simulink model "MultiVehicleModel"  (R2014a)
settings: Solver=ode1  StartTime=0.0  StopTime=inf  FixedStep=simPars.SampleTime  RelTol=1e-3
undefined symbols (not defined in the file or in its folder): DiscIntNeverNeededParam, Earth, Env, eul_0, FWFleet, GVFleet, m, RCFleet, s, WGS84
undefined symbols (not defined in the file): simPars
libraries: simulink x26, aerolibtransform2 x7, instrumentlib x6, Actuator_Lib x5, aerolib6dofsys x4, etargetslib x3, aerolibasang x3, aerolibconvert2 x2, aerolibutil x1, aerolibatmos2 x1, aerolibobsolete x1, aerolibgravity2 x1
(part 3 of 4)

== system MultiVehicleModel/Reconnaissance Fleet/UMN - Uninhabited Aerial Vehicle Fleet/Nonlinear UAV Model/Environment ==
  States : Inport
  Bus Creator : BusCreator  Inputs=9
  Bus Selector1 : BusSelector  OutputSignals=Nav.Alt (Above Mean Sea Level) [m]
  Bus Selector2 : BusSelector  OutputSignals=Nav.Altitude [m],Nav.Geodetic Latitude [deg],Nav.Geodetic Longitude [deg]
  Bus Selector3 : BusSelector  OutputSignals=Nav.Geodetic Latitude [deg],Nav.Geodetic Longitude [deg],Nav.Altitude [m]  OutputAsBus=on
  Bus Selector4 : BusSelector  OutputSignals=WindAxesParam.V_s [m/s],R_be [3x3],Nav.Alt (Above Ground Level) [m]
  COESA Atmosphere Model : aerolibatmos2/COESA Atmosphere Model  units=Metric (MKS)  spec=1976 COESA-extended U.S. Standard Atmosphere  model=Profile  profile_var=High temperature  profile_percent=1%  profile_alt=5 km (16404 ft)  envelope_var=High temperature  envelope_percent=1%  action=Warning
  Constant : Constant  Value=Env.DecimalYear
  Magnetic Model : Subsystem  BlockChoice=WMM 2005
      settings: AttributesFormatString=%<BlockChoice>  TemplateBlock=Environment_Lib/Magnetic Model  MemberBlocks=WMM 2005,WMM Bypass
  README : simulink/Model-Wide Utilities/DocBlock  DocumentType=Text
      content=|
      | Environment Model
      |
      | This block uses the Aerospace Blockset models for Earth's atmosphere,
      | gravity, magnetic field, and wind.
      |
      | The atmosphere is modeled using the 1976 Standard Atmosphere block.
      |
      | Winds are modeled in two portions: steady and unsteady. The steady
      | portion is defined by a speed and direction, and is horizontal only. The
      | unsteady portion is made up of a wind gust model and a turbulence model.
      |
      | The Dryden Wind Turbulence Model is used to model turbulence. The
      | intensity of the turbulence at low altitude (<1000ft) is determined by
      | the wind speed and direction; this is set as separate variables from the
      | steady wind speed and direction. The turbulence is off by default, and
      | can be enabled by setting the Env.Winds.TurbulenceOn boolean in
      | UAV_config.m.
      |
      | The Discrete Gust Model is used to model wind gusts. Parameters are time
      | on, duration (length), and amplitude, in three axes (u,v,w). These
      | parameters are set in Env.Winds, in UAV_config.m
      |
      | Note the booleans in the Env.Winds stucture to turn on each wind
      | component: >> Env.Winds
      |
      | ans =
      |
      |      TurbulenceOn: 0
      |     TurbWindSpeed: 0
      |       TurbWindDir: 0
      |            GustOn: 0
      |     GustStartTime: 0
      |        GustLength: [1 1 1]
      |     GustAmplitude: [1 1 1]
      |      SteadyWindOn: 0
      |         WindSpeed: 0
      |           WindDir: 0
      |
      |
      | The WGS84 Gravity Model is used to model Earth's gravity as a function of
      | latitude, longitude, and altitude.
      |
      | The World Magnetic Model 2005 is used to model Earth's magnetic field as
      | a function of latitude, longitude, and altitude. The current decimal year
      | is input.
      |
      | *Note for trim/linearizing: the Dryden turbulence model and the World
      | Magnetic Model 2005 have many internal states, which makes trimming and
      | linearizing difficult. Thus "Bypass" blocks are substituted for the Winds
      | and Magnetic Model blocks using Configurable Subsystems. For the
      | UAV_NL.mdl, the block choices are automatically set to "Bypass" using the
      | models "InitFcn" callback, which can be viewed by using the Model
      | Explorer, selecting UAV_NL, and going to the "Callbacks" tab. The Nonlinear
      | UAV Model block will then show up as a Parameterized Link (red arrow in the
      | lower left corner). The SIL and PIL sims use the default blocks, and should
      | have a normal library link (black arrow).
  "WGS84 Gravity Model " : aerolibgravity2/WGS84 Gravity Model   model=WGS84 Taylor Series  units=Metric (MKS)  no_atmos=on  precessing=on  jd_loc=off  month=October  day=10  year=2004  no_centrifugal=on  action=Warning
  Winds : Subsystem  BlockChoice=Wind & Turbulence
      settings: AttributesFormatString=%<BlockChoice>  TemplateBlock=Environment_Lib/Winds  MemberBlocks=Wind & Turbulence,Wind Bypass
  EnvData : Outport
  wires:
  Constant/1 -> Magnetic Model/4(Decimal Year)
  Bus Selector3/1 -> "WGS84 Gravity Model "/1
  Bus Selector2/3 -> Magnetic Model/3(Longitude)  "<Geodetic Longitude [deg]>"
  Bus Selector2/2 -> Magnetic Model/2(Latitude)  "<Geodetic Latitude [deg]>"
  Bus Selector2/1 -> Magnetic Model/1(Altitude)  "<Altitude [m]>"
  Magnetic Model/1(Magnetic Field) -> Bus Creator/9  "Magnetic Field [nT]"
  "WGS84 Gravity Model "/1 -> Bus Creator/8  "Gravity [m/s^2]"
  Winds/3(WindAngVel [rad/s]) -> Bus Creator/7  "WindAngVel [rad/s]"
  Winds/2(WindGust [m/s]) -> Bus Creator/6  "WindGust [m/s]"
  Winds/1(SteadyWind [m/s]) -> Bus Creator/5  "SteadyWind [m/s]"
  COESA Atmosphere Model/4 -> Bus Creator/4  "Density [kg/m^3]"
  COESA Atmosphere Model/1 -> Bus Creator/1  "Temperature [K]"
  COESA Atmosphere Model/2 -> Bus Creator/2  "Speed of Sound [m/s]"
  COESA Atmosphere Model/3 -> Bus Creator/3  "Pressure [Pa]"
  States/1 -> Bus Selector1/1, Bus Selector2/1, Bus Selector3/1, Bus Selector4/1
  Bus Selector1/1 -> COESA Atmosphere Model/1  "<Alt (Above Mean Sea Level) [m]>"
  Bus Creator/1 -> EnvData/1
  Bus Selector4/1 -> Winds/1(V_s [m/s])  "<V_s [m/s]>"
  Bus Selector4/2 -> Winds/2(R_be [3x3])  "<R_be [3x3]>"
  Bus Selector4/3 -> Winds/3(h (m))  "<Alt (Above Ground Level) [m]>"

== system MultiVehicleModel/Reconnaissance Fleet/UMN - Uninhabited Aerial Vehicle Fleet/Nonlinear UAV Model/Forces and Moments ==
  Control Inputs : Inport
  States : Inport  Port=2
  EnvData : Inport  Port=3
  Aerodynamic Forces and Moments : Subsystem  AncestorBlock=Aero_Lib/Aerodynamic Forces and Moments
      mask help:
      | Set the boolean Aero Model Selection flag to 1 to use the FASER aerodynamic
      | model; otherwise, the Ultra Stick aero model will be used.
      |
      | This is done in this block's Mask Initialization commands. Also set is the
      | axes input for computing the forces and moments from the coefficients.
  Bus Selector1 : BusSelector  OutputSignals=throttle [nd]
  Control Inputs1 : InportShadow
  Electric Propulsion Forces and Moments : Propulsion_Lib/Electric Propulsion Forces and Moments
  "Gravitational Force " : Gravity_Lib/Gravitational Force 
  README : simulink/Model-Wide Utilities/DocBlock  DocumentType=Text
      content=|
      | Forces and Moments
      |
      | This block models all of the relevant external forces and
      | moments acting on the aircraft. The Aerodynamic Forces and Moments block
      | contains the aero models, and is a masked subsystem. The input parameter to
      | this block is a boolean which controls which aero model (either FASER or
      | the Ultrastick) is used.
      |
      | The Gravitational Force block models the effect of Earth's graviy field on
      | the aircraft.
      |
      | The Electric Propulsion Forces and Moments block contains the electric
      | motor model.
      |
      | Note the non-gravitational forces (nonGravForces) are output- this is what
      | an accelerometer on the aircraft would measure, and is used in the sensor
      | models.
  Sum : Sum  Inputs=+++
  Sum1 : Sum  Inputs=|++
  Sum2 : Sum  Inputs=|++
  Total Force : Outport
  Total Moment : Outport  Port=2
  nonGravForces : Outport  Port=3
  wires:
  Bus Selector1/1 -> Electric Propulsion Forces and Moments/3  "<throttle [nd]>"
  Control Inputs/1 -> Aerodynamic Forces and Moments/1(Control Surfaces)
  States/1 -> Aerodynamic Forces and Moments/2(States), "Gravitational Force "/2, Electric Propulsion Forces and Moments/2
  EnvData/1 -> Aerodynamic Forces and Moments/3(EnvData), "Gravitational Force "/1, Electric Propulsion Forces and Moments/1
  Control Inputs1/1 -> Bus Selector1/1
  Aerodynamic Forces and Moments/2(F_aero_body) -> Sum/1, Sum2/1
  "Gravitational Force "/1 -> Sum/2
  Electric Propulsion Forces and Moments/1 -> Sum2/2, Sum/3
  Sum/1 -> Total Force/1
  Aerodynamic Forces and Moments/1(M_aero_body) -> Sum1/1
  Electric Propulsion Forces and Moments/2 -> Sum1/2
  Sum1/1 -> Total Moment/1
  Sum2/1 -> nonGravForces/1

== system MultiVehicleModel/Reconnaissance Fleet/UMN - Uninhabited Aerial Vehicle Fleet/Nonlinear UAV Model/Packaging initial Euler angles  ==
  Position and heading : Inport
  Constant : Constant  Value=AC.TrimCondition.AttitudeIni(1:2)
  Demux9 : Demux  Outputs=[3 1]
  Mux : Mux  Inputs=[2 1]
  T : Terminator
  Initial Euler angles : Outport
  wires:
  Position and heading/1 -> Demux9/1
  Mux/1 -> Initial Euler angles/1
  Demux9/1 -> T/1
  Demux9/2 -> Mux/2
  Constant/1 -> Mux/1

== system MultiVehicleModel/Reconnaissance Fleet/UMN - Uninhabited Aerial Vehicle Fleet/Sensors/NoiseModel ==
  In1 : Inport
  Add : Sum  Inputs=+++
  Band-Limited White Noise : simulink/Sources/Band-Limited White Noise  Cov=sigma  Ts=timestep  seed=seed
  Gain : Gain  Gain=scf
  Gear1 : Constant  Value=bias
  Gear2 : Constant  Value=noise_on
  Noise_on : Switch  Threshold=0.5  SaturateOnIntegerOverflow=on  InputSameDT=on
  Out1 : Outport
  wires:
  In1/1 -> Gain/1, Noise_on/3
  Gain/1 -> Add/3
  Gear1/1 -> Add/2
  Add/1 -> Noise_on/1
  Band-Limited White Noise/1 -> Add/1
  Gear2/1 -> Noise_on/2
  Noise_on/1 -> Out1/1

== system MultiVehicleModel/Reconnaissance Fleet/UMN - Uninhabited Aerial Vehicle Fleet/Sensors/NoiseModel1 ==
  In1 : Inport
  Add : Sum  Inputs=+++
  Band-Limited White Noise : simulink/Sources/Band-Limited White Noise  Cov=sigma  Ts=timestep  seed=seed
  Gain : Gain  Gain=scf
  Gear1 : Constant  Value=bias
  Gear2 : Constant  Value=noise_on
  Noise_on : Switch  Threshold=0.5  SaturateOnIntegerOverflow=on  InputSameDT=on
  Out1 : Outport
  wires:
  In1/1 -> Gain/1, Noise_on/3
  Gain/1 -> Add/3
  Gear1/1 -> Add/2
  Add/1 -> Noise_on/1
  Band-Limited White Noise/1 -> Add/1
  Gear2/1 -> Noise_on/2
  Noise_on/1 -> Out1/1

== system MultiVehicleModel/Reconnaissance Fleet/UMN - Uninhabited Aerial Vehicle Fleet/Sensors/NoiseModel10 ==
  In1 : Inport
  Add : Sum  Inputs=+++
  Band-Limited White Noise : simulink/Sources/Band-Limited White Noise  Cov=sigma  Ts=timestep  seed=seed
  Gain : Gain  Gain=scf
  Gear1 : Constant  Value=bias
  Gear2 : Constant  Value=noise_on
  Noise_on : Switch  Threshold=0.5  SaturateOnIntegerOverflow=on  InputSameDT=on
  Out1 : Outport
  wires:
  In1/1 -> Gain/1, Noise_on/3
  Gain/1 -> Add/3
  Gear1/1 -> Add/2
  Add/1 -> Noise_on/1
  Band-Limited White Noise/1 -> Add/1
  Gear2/1 -> Noise_on/2
  Noise_on/1 -> Out1/1

== system MultiVehicleModel/Reconnaissance Fleet/UMN - Uninhabited Aerial Vehicle Fleet/Sensors/NoiseModel11 ==
  In1 : Inport
  Add : Sum  Inputs=+++
  Band-Limited White Noise : simulink/Sources/Band-Limited White Noise  Cov=sigma  Ts=timestep  seed=seed
  Gain : Gain  Gain=scf
  Gear1 : Constant  Value=bias
  Gear2 : Constant  Value=noise_on
  Noise_on : Switch  Threshold=0.5  SaturateOnIntegerOverflow=on  InputSameDT=on
  Out1 : Outport
  wires:
  In1/1 -> Gain/1, Noise_on/3
  Gain/1 -> Add/3
  Gear1/1 -> Add/2
  Add/1 -> Noise_on/1
  Band-Limited White Noise/1 -> Add/1
  Gear2/1 -> Noise_on/2
  Noise_on/1 -> Out1/1

== system MultiVehicleModel/Reconnaissance Fleet/UMN - Uninhabited Aerial Vehicle Fleet/Sensors/NoiseModel12 ==
  In1 : Inport
  Add : Sum  Inputs=+++
  Band-Limited White Noise : simulink/Sources/Band-Limited White Noise  Cov=sigma  Ts=timestep  seed=seed
  Gain : Gain  Gain=scf
  Gear1 : Constant  Value=bias
  Gear2 : Constant  Value=noise_on
  Noise_on : Switch  Threshold=0.5  SaturateOnIntegerOverflow=on  InputSameDT=on
  Out1 : Outport
  wires:
  In1/1 -> Gain/1, Noise_on/3
  Gain/1 -> Add/3
  Gear1/1 -> Add/2
  Add/1 -> Noise_on/1
  Band-Limited White Noise/1 -> Add/1
  Gear2/1 -> Noise_on/2
  Noise_on/1 -> Out1/1

== system MultiVehicleModel/Reconnaissance Fleet/UMN - Uninhabited Aerial Vehicle Fleet/Sensors/NoiseModel2 ==
  In1 : Inport
  Add : Sum  Inputs=+++
  Band-Limited White Noise : simulink/Sources/Band-Limited White Noise  Cov=sigma  Ts=timestep  seed=seed
  Gain : Gain  Gain=scf
  Gear1 : Constant  Value=bias
  Gear2 : Constant  Value=noise_on
  Noise_on : Switch  Threshold=0.5  SaturateOnIntegerOverflow=on  InputSameDT=on
  Out1 : Outport
  wires:
  In1/1 -> Gain/1, Noise_on/3
  Gain/1 -> Add/3
  Gear1/1 -> Add/2
  Add/1 -> Noise_on/1
  Band-Limited White Noise/1 -> Add/1
  Gear2/1 -> Noise_on/2
  Noise_on/1 -> Out1/1

== system MultiVehicleModel/Reconnaissance Fleet/UMN - Uninhabited Aerial Vehicle Fleet/Sensors/NoiseModel3 ==
  In1 : Inport
  Add : Sum  Inputs=+++
  Band-Limited White Noise : simulink/Sources/Band-Limited White Noise  Cov=sigma  Ts=timestep  seed=seed
  Gain : Gain  Gain=scf
  Gear1 : Constant  Value=bias
  Gear2 : Constant  Value=noise_on
  Noise_on : Switch  Threshold=0.5  SaturateOnIntegerOverflow=on  InputSameDT=on
  Out1 : Outport
  wires:
  In1/1 -> Gain/1, Noise_on/3
  Gain/1 -> Add/3
  Gear1/1 -> Add/2
  Add/1 -> Noise_on/1
  Band-Limited White Noise/1 -> Add/1
  Gear2/1 -> Noise_on/2
  Noise_on/1 -> Out1/1

== system MultiVehicleModel/Reconnaissance Fleet/UMN - Uninhabited Aerial Vehicle Fleet/Sensors/NoiseModel4 ==
  In1 : Inport
  Add : Sum  Inputs=+++
  Band-Limited White Noise : simulink/Sources/Band-Limited White Noise  Cov=sigma  Ts=timestep  seed=seed
  Gain : Gain  Gain=scf
  Gear1 : Constant  Value=bias
  Gear2 : Constant  Value=noise_on
  Noise_on : Switch  Threshold=0.5  SaturateOnIntegerOverflow=on  InputSameDT=on
  Out1 : Outport
  wires:
  In1/1 -> Gain/1, Noise_on/3
  Gain/1 -> Add/3
  Gear1/1 -> Add/2
  Add/1 -> Noise_on/1
  Band-Limited White Noise/1 -> Add/1
  Gear2/1 -> Noise_on/2
  Noise_on/1 -> Out1/1

== system MultiVehicleModel/Reconnaissance Fleet/UMN - Uninhabited Aerial Vehicle Fleet/Sensors/NoiseModel5 ==
  In1 : Inport
  Add : Sum  Inputs=+++
  Band-Limited White Noise : simulink/Sources/Band-Limited White Noise  Cov=sigma  Ts=timestep  seed=seed
  Gain : Gain  Gain=scf
  Gear1 : Constant  Value=bias
  Gear2 : Constant  Value=noise_on
  Noise_on : Switch  Threshold=0.5  SaturateOnIntegerOverflow=on  InputSameDT=on
  Out1 : Outport
  wires:
  In1/1 -> Gain/1, Noise_on/3
  Gain/1 -> Add/3
  Gear1/1 -> Add/2
  Add/1 -> Noise_on/1
  Band-Limited White Noise/1 -> Add/1
  Gear2/1 -> Noise_on/2
  Noise_on/1 -> Out1/1

== system MultiVehicleModel/Reconnaissance Fleet/UMN - Uninhabited Aerial Vehicle Fleet/Sensors/NoiseModel6 ==
  In1 : Inport
  Add : Sum  Inputs=+++
  Band-Limited White Noise : simulink/Sources/Band-Limited White Noise  Cov=sigma  Ts=timestep  seed=seed
  Gain : Gain  Gain=scf
  Gear1 : Constant  Value=bias
  Gear2 : Constant  Value=noise_on
  Noise_on : Switch  Threshold=0.5  SaturateOnIntegerOverflow=on  InputSameDT=on
  Out1 : Outport
  wires:
  In1/1 -> Gain/1, Noise_on/3
  Gain/1 -> Add/3
  Gear1/1 -> Add/2
  Add/1 -> Noise_on/1
  Band-Limited White Noise/1 -> Add/1
  Gear2/1 -> Noise_on/2
  Noise_on/1 -> Out1/1

== system MultiVehicleModel/Reconnaissance Fleet/UMN - Uninhabited Aerial Vehicle Fleet/Sensors/NoiseModel7 ==
  In1 : Inport
  Add : Sum  Inputs=+++
  Band-Limited White Noise : simulink/Sources/Band-Limited White Noise  Cov=sigma  Ts=timestep  seed=seed
  Gain : Gain  Gain=scf
  Gear1 : Constant  Value=bias
  Gear2 : Constant  Value=noise_on
  Noise_on : Switch  Threshold=0.5  SaturateOnIntegerOverflow=on  InputSameDT=on
  Out1 : Outport
  wires:
  In1/1 -> Gain/1, Noise_on/3
  Gain/1 -> Add/3
  Gear1/1 -> Add/2
  Add/1 -> Noise_on/1
  Band-Limited White Noise/1 -> Add/1
  Gear2/1 -> Noise_on/2
  Noise_on/1 -> Out1/1

== system MultiVehicleModel/Reconnaissance Fleet/UMN - Uninhabited Aerial Vehicle Fleet/Sensors/NoiseModel8 ==
  In1 : Inport
  Add : Sum  Inputs=+++
  Band-Limited White Noise : simulink/Sources/Band-Limited White Noise  Cov=sigma  Ts=timestep  seed=seed
  Gain : Gain  Gain=scf
  Gear1 : Constant  Value=bias
  Gear2 : Constant  Value=noise_on
  Noise_on : Switch  Threshold=0.5  SaturateOnIntegerOverflow=on  InputSameDT=on
  Out1 : Outport
  wires:
  In1/1 -> Gain/1, Noise_on/3
  Gain/1 -> Add/3
  Gear1/1 -> Add/2
  Add/1 -> Noise_on/1
  Band-Limited White Noise/1 -> Add/1
  Gear2/1 -> Noise_on/2
  Noise_on/1 -> Out1/1

== system MultiVehicleModel/Reconnaissance Fleet/UMN - Uninhabited Aerial Vehicle Fleet/Sensors/NoiseModel9 ==
  In1 : Inport
  Add : Sum  Inputs=+++
  Band-Limited White Noise : simulink/Sources/Band-Limited White Noise  Cov=sigma  Ts=timestep  seed=seed
  Gain : Gain  Gain=scf
  Gear1 : Constant  Value=bias
  Gear2 : Constant  Value=noise_on
  Noise_on : Switch  Threshold=0.5  SaturateOnIntegerOverflow=on  InputSameDT=on
  Out1 : Outport
  wires:
  In1/1 -> Gain/1, Noise_on/3
  Gain/1 -> Add/3
  Gear1/1 -> Add/2
  Add/1 -> Noise_on/1
  Band-Limited White Noise/1 -> Add/1
  Gear2/1 -> Noise_on/2
  Noise_on/1 -> Out1/1

== system MultiVehicleModel/Rotorcraft fleet/Multiple Rotorcraft/Guidance /From geodetic to NED coordinate representation ==
  geodetic [lat,lon,alt] : Inport  Partition=on  PartitionDimension=2  PartitionWidth=1
  Demux : Demux  Outputs=[2 1]
  For Each : ForEach  DisableCoverage=on  IndexMode=One-based
  Ground Height1 : Constant  Value=Env.GroundAlt
  LLA to Flat Earth : aerolibtransform2/LLA to Flat Earth  units=Metric (MKS)  ptype=Earth (WGS84)  F=1/298.257223563  R=6378137  LL0=RCFleet.IC.geodetic(1:2)  psi=0
  "[N,E,D] (m)" : Outport  ConcatenationDimension=2
  wires:
  LLA to Flat Earth/1 -> "[N,E,D] (m)"/1
  Demux/1 -> LLA to Flat Earth/1
  Demux/2 -> LLA to Flat Earth/2
  geodetic [lat,lon,alt]/1 -> Demux/1
  Ground Height1/1 -> LLA to Flat Earth/3

== system MultiVehicleModel/Rotorcraft fleet/Multiple Rotorcraft/Navigation/EGM-96 Geoid Model ==
  Position : Inport
  Demux2 : Demux  Outputs=3
  Look-Up Table (2-D) : Lookup2D  RowIndex=Lat  ColumnIndex=Lon  Table=Alterr'  SaturateOnIntegerOverflow=on  InputSameDT=on
  Sum : Sum  Inputs=|+++
  WGS-84 correction : Constant  Value=-0.53
  MSLAlt : Outport
  wires:
  Demux2/2 -> Look-Up Table (2-D)/2
  Demux2/1 -> Look-Up Table (2-D)/1
  Position/1 -> Demux2/1
  Demux2/3 -> Sum/2
  Sum/1 -> MSLAlt/1
  Look-Up Table (2-D)/1 -> Sum/1
  WGS-84 correction/1 -> Sum/3

== system MultiVehicleModel/Rotorcraft fleet/Multiple Rotorcraft/Navigation/Ground Detection ==
  MSLAlt : Inport
  GndAlt : Inport  Port=2
  False : Constant  Value=0
  Sum : Sum  Inputs=|+-  SaturateOnIntegerOverflow=on  InputSameDT=on  OutDataTypeStr=Inherit: Same as first input
  Switch : Switch  SaturateOnIntegerOverflow=on  InputSameDT=on
  True : Constant
  AConGnd : Outport
  AGLAlt : Outport  Port=2
  wires:
  MSLAlt/1 -> Sum/1
  GndAlt/1 -> Sum/2
  Sum/1 -> Switch/2, AGLAlt/1
  False/1 -> Switch/1
  True/1 -> Switch/3
  Switch/1 -> AConGnd/1

== system MultiVehicleModel/Rotorcraft fleet/Multiple Rotorcraft/Navigation/Latitude Bound [-180,180] ==
  In : Inport
  2pi : Constant  Value=360
  Math Function : Math  Operator=mod  SaturateOnIntegerOverflow=on
  Sum1 : Sum  Inputs=|+-  SaturateOnIntegerOverflow=on  InputSameDT=on  OutDataTypeStr=Inherit: Same as first input
  Sum2 : Sum  Inputs=|++  SaturateOnIntegerOverflow=on  InputSameDT=on  OutDataTypeStr=Inherit: Same as first input
  pi : Constant  Value=180
  Out : Outport
  wires:
  Math Function/1 -> Sum1/1
  2pi/1 -> Math Function/2
  In/1 -> Sum2/1
  Sum2/1 -> Math Function/1
  pi/1 -> Sum2/2, Sum1/2
  Sum1/1 -> Out/1

== system MultiVehicleModel/Rotorcraft fleet/Multiple Rotorcraft/Navigation/Longitude Bound 0-360 ==
  In : Inport
  2pi : Constant  Value=360
  Math Function : Math  Operator=mod  SaturateOnIntegerOverflow=on
  Out : Outport
  wires:
  Math Function/1 -> Out/1
  2pi/1 -> Math Function/2
  In/1 -> Math Function/1

== system MultiVehicleModel/Reconnaissance Fleet/UMN - Uninhabited Aerial Vehicle Fleet/Control System/Control_Algorithm /Altitude Tracker ==
  h_cmd [m/s] : Inport
  h [m] : Inport  Port=2
  Altitude Tracker : Subsystem
  Discrete Transfer Fcn : DiscreteTransferFcn  Numerator=[control.LP_filter(1,2)]  Denominator=[1 control.LP_filter(2,2)]  InitialStates=OperatingPoint.op_report.Outputs(4).y/control.LP_filter(1,2)  SampleTime=SampleTime
  Saturation : Saturate  UpperLimit=control.theta_sat*pi/180  LowerLimit=-control.theta_sat*pi/180  SampleTime=SampleTime
  Sum4 : Sum  Inputs=|+-  SampleTime=SampleTime
  Sum5 : Sum  Inputs=|+-  SampleTime=SampleTime
  trim altitude : Constant  Value=OperatingPoint.op_report.Outputs(4).y
  theta_cmd [rad] : Outport
  wires:
  h_cmd [m/s]/1 -> Sum4/1
  trim altitude/1 -> Sum5/2
  Sum5/1 -> Sum4/2
  h [m]/1 -> Discrete Transfer Fcn/1
  Discrete Transfer Fcn/1 -> Sum5/1
  Sum4/1 -> Altitude Tracker/2(error)
  Altitude Tracker/1(h_out) -> Saturation/1, Altitude Tracker/1(" h_out")
  Saturation/1 -> theta_cmd [rad]/1

== system MultiVehicleModel/Reconnaissance Fleet/UMN - Uninhabited Aerial Vehicle Fleet/Control System/Control_Algorithm /Velocity Tracker ==
  V_cmd [m/s] : Inport
  V_s [m/s] : Inport  Port=2
  "    " : Constant  Value=TrimCondition.WindAxesIni(1)
  Anti Windup : Actuator_Lib/Anti Windup  MAX_DEF=AC.Actuator.throttle.PosLim-TrimCondition.Inputs.throttle  MIN_DEF=AC.Actuator.throttle.NegLim-TrimCondition.Inputs.throttle  gain_sign=on
  Discrete Transfer Fcn : DiscreteTransferFcn  Numerator=[control.LP_filter(1,2)]  Denominator=[1 control.LP_filter(2,2)]  InitialStates=TrimCondition.target.V_s/control.LP_filter(1,2)  SampleTime=SampleTime
  Discrete-Time Integrator : DiscreteIntegrator  SampleTime=.02  ICPrevOutput=DiscIntNeverNeededParam  ICPrevScaledInput=DiscIntNeverNeededParam
  Gain : Gain  Gain=control.kp_VT
  Gain1 : Gain  Gain=control.ki_VT
  Saturation1 : Saturate  UpperLimit=AC.Actuator.throttle.PosLim-TrimCondition.Inputs.throttle  LowerLimit=AC.Actuator.throttle.NegLim-TrimCondition.Inputs.throttle  SampleTime=SampleTime
  Sum : Sum  Inputs=|++
  Sum1 : Sum  Inputs=|+-
  Sum5 : Sum  Inputs=|+-  SampleTime=SampleTime
  "Throttle " : Outport
  wires:
  Discrete-Time Integrator/1 -> Gain1/1
  Gain1/1 -> Sum/1
  Gain/1 -> Sum/2
  V_cmd [m/s]/1 -> Sum1/1
  Sum/1 -> Saturation1/1, Anti Windup/1
  "    "/1 -> Sum5/2
  Sum5/1 -> Sum1/2
  V_s [m/s]/1 -> Discrete Transfer Fcn/1
  Saturation1/1 -> "Throttle "/1
  Sum1/1 -> Anti Windup/2, Gain/1
  Anti Windup/1 -> Discrete-Time Integrator/1
  Discrete Transfer Fcn/1 -> Sum5/1

== system MultiVehicleModel/Reconnaissance Fleet/UMN - Uninhabited Aerial Vehicle Fleet/Control System/Control_Algorithm /baseline control ==
  theta_cmd [rad] : Inport
  theta [rad] : Inport  Port=2
  q [rad/sec] : Inport  Port=3
  r [rad/sec] : Inport  Port=4
  phi_cmd [rad] : Inport  Port=5
  phi [rad] : Inport  Port=6
  p [rad/sec] : Inport  Port=7
  Phi Tracker : Subsystem
  Theta Tracker : Subsystem
  Yaw Damper : Subsystem
  elevator [rad] : Outport
  rudder [rad] : Outport  Port=2
  aileron [rad] : Outport  Port=3
  wires:
  p [rad/sec]/1 -> Phi Tracker/3(p [rad])
  phi [rad]/1 -> Phi Tracker/2(phi [rad])
  phi_cmd [rad]/1 -> Phi Tracker/1(phi_cmd [rad])
  Phi Tracker/1(aileron [rad]) -> aileron [rad]/1
  r [rad/sec]/1 -> Yaw Damper/1(r [rad/sec])
  Yaw Damper/1(rudder [rad]) -> rudder [rad]/1
  Theta Tracker/1(elevator [rad]) -> elevator [rad]/1
  q [rad/sec]/1 -> Theta Tracker/3(q [rad/sec])
  theta [rad]/1 -> Theta Tracker/2(theta [rad])
  theta_cmd [rad]/1 -> Theta Tracker/1(theta_cmd [rad/s])

== system MultiVehicleModel/Reconnaissance Fleet/UMN - Uninhabited Aerial Vehicle Fleet/Control System/Control_Algorithm /ground trak angle control law ==
  ground track reference angle (rad) : Inport
  heading angle (rad) : Inport  Port=2
  Saturation : Saturate  UpperLimit=40*pi/180  LowerLimit=-40*pi/180
  Sum : Sum  Inputs=|+-
  normalize angle between pi and -pi (rad) : MATLAB Function  TreatAsAtomicUnit=on
  proportional control : Gain
  phi cmd (rad) : Outport
  wires:
  ground track reference angle (rad)/1 -> Sum/1
  normalize angle between pi and -pi (rad)/1(angleOut) -> proportional control/1
  heading angle (rad)/1 -> Sum/2
  Sum/1 -> normalize angle between pi and -pi (rad)/1(angleIn)
  Saturation/1 -> phi cmd (rad)/1
  proportional control/1 -> Saturation/1

== system MultiVehicleModel/Reconnaissance Fleet/UMN - Uninhabited Aerial Vehicle Fleet/Guidance algorithm/From geodetic to NED coordinate representation/EGM-96 Geoid Model ==
  Position : Inport
  Demux2 : Demux  Outputs=3
  Look-Up Table (2-D) : Lookup2D  RowIndex=Lat  ColumnIndex=Lon  Table=Alterr'  SaturateOnIntegerOverflow=on  InputSameDT=on
  Sum : Sum  Inputs=|+++
  WGS-84 correction : Constant  Value=-0.53
  MSLAlt : Outport
  wires:
  Demux2/2 -> Look-Up Table (2-D)/2
  Demux2/1 -> Look-Up Table (2-D)/1
  Position/1 -> Demux2/1
  Demux2/3 -> Sum/2
  Sum/1 -> MSLAlt/1
  Look-Up Table (2-D)/1 -> Sum/1
  WGS-84 correction/1 -> Sum/3

== system MultiVehicleModel/Reconnaissance Fleet/UMN - Uninhabited Aerial Vehicle Fleet/Guidance algorithm/From geodetic to NED coordinate representation/Ground Detection ==
  MSLAlt : Inport
  GndAlt : Inport  Port=2
  False : Constant  Value=0
  Sum : Sum  Inputs=|+-  SaturateOnIntegerOverflow=on  InputSameDT=on  OutDataTypeStr=Inherit: Same as first input
  Switch : Switch  SaturateOnIntegerOverflow=on  InputSameDT=on
  True : Constant
  AConGnd : Outport
  AGLAlt : Outport  Port=2
  wires:
  MSLAlt/1 -> Sum/1
  GndAlt/1 -> Sum/2
  Sum/1 -> Switch/2, AGLAlt/1
  False/1 -> Switch/1
  True/1 -> Switch/3
  Switch/1 -> AConGnd/1

== system MultiVehicleModel/Reconnaissance Fleet/UMN - Uninhabited Aerial Vehicle Fleet/Guidance algorithm/From geodetic to NED coordinate representation/Latitude Bound [-180,180] ==
  In : Inport
  2pi : Constant  Value=360
  Math Function : Math  Operator=mod  SaturateOnIntegerOverflow=on
  Sum1 : Sum  Inputs=|+-  SaturateOnIntegerOverflow=on  InputSameDT=on  OutDataTypeStr=Inherit: Same as first input
  Sum2 : Sum  Inputs=|++  SaturateOnIntegerOverflow=on  InputSameDT=on  OutDataTypeStr=Inherit: Same as first input
  pi : Constant  Value=180
  Out : Outport
  wires:
  Math Function/1 -> Sum1/1
  2pi/1 -> Math Function/2
  In/1 -> Sum2/1
  Sum2/1 -> Math Function/1
  pi/1 -> Sum2/2, Sum1/2
  Sum1/1 -> Out/1

== system MultiVehicleModel/Reconnaissance Fleet/UMN - Uninhabited Aerial Vehicle Fleet/Guidance algorithm/From geodetic to NED coordinate representation/Longitude Bound 0-360 ==
  In : Inport
  2pi : Constant  Value=360
  Math Function : Math  Operator=mod  SaturateOnIntegerOverflow=on
  Out : Outport
  wires:
  Math Function/1 -> Out/1
  2pi/1 -> Math Function/2
  In/1 -> Math Function/1

== system MultiVehicleModel/Reconnaissance Fleet/UMN - Uninhabited Aerial Vehicle Fleet/Nonlinear UAV Model/6DoF EOM/calculate DCM and Euler angles ==
  "p q r " : Inport
  euler ini. (rad) : Inport  Port=2
  Rotation Angles to Direction Cosine Matrix : aerolibtransform2/Rotation Angles to Direction Cosine Matrix  rotationOrder=ZYX
  Selector : Selector  InputPortWidth=3  Indices=[3 2 1]
  phi theta psi : Integrator  InitialConditionSource=external  InitialCondition=eul_0
  phidot thetadot psidot : aerolib6dofsys/DCM & Euler Angles (Euler)/phidot thetadot psidot
  DCM1 : Outport
  Euler1 : Outport  Port=2
  wires:
  Selector/1 -> Rotation Angles to Direction Cosine Matrix/1
  phidot thetadot psidot/1 -> phi theta psi/1
  phi theta psi/1 -> Selector/1, Euler1/1, phidot thetadot psidot/2
  Rotation Angles to Direction Cosine Matrix/1 -> DCM1/1
  "p q r "/1 -> phidot thetadot psidot/1
  euler ini. (rad)/1 -> phi theta psi/2

== system MultiVehicleModel/Reconnaissance Fleet/UMN - Uninhabited Aerial Vehicle Fleet/Nonlinear UAV Model/6DoF EOM/transform to Inertial axes  ==
  x y z : Inport
  transform coefficients : Inport  Port=2
  Product : Product  Multiplication=Matrix(*)  SaturateOnIntegerOverflow=on  InputSameDT=on  OutDataTypeStr=Inherit: Same as first input
  Reshape1 : Reshape  OutputDimensionality=Column vector (2-D)
  Reshape2 : Reshape
  Ve : Outport
  wires:
  Product/1 -> Reshape2/1
  transform coefficients/1 -> Product/1
  x y z/1 -> Reshape1/1
  Reshape1/1 -> Product/2
  Reshape2/1 -> Ve/1

== system MultiVehicleModel/Reconnaissance Fleet/UMN - Uninhabited Aerial Vehicle Fleet/Nonlinear UAV Model/Auxiliary Equations/Euler Angle Bounds ==
  Euler_nobound : Inport
  2pi Bound : Subsystem
  Demux : Demux  Outputs=3
  Mux : Mux  Inputs=3
  pi Bound : Subsystem
  pi/2 Bound : Subsystem
  Euler_bound : Outport
  wires:
  2pi Bound/1(Out) -> Mux/3
  Demux/3 -> 2pi Bound/1(In)
  Demux/2 -> pi Bound/1(In)
  Demux/1 -> pi/2 Bound/1(In)
  Euler_nobound/1 -> Demux/1
  Mux/1 -> Euler_bound/1
  pi/2 Bound/1(Out) -> Mux/1
  pi Bound/1(Out) -> Mux/2

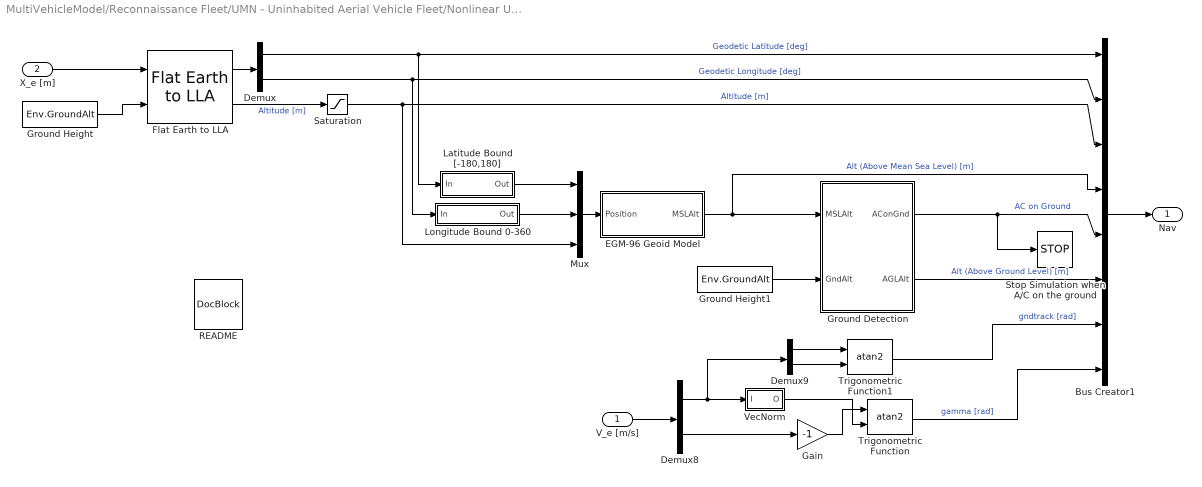
== system MultiVehicleModel/Reconnaissance Fleet/UMN - Uninhabited Aerial Vehicle Fleet/Nonlinear UAV Model/Auxiliary Equations/Navigation ==
  V_e [m/s] : Inport
  X_e [m] : Inport  Port=2
  Bus Creator1 : BusCreator  Inputs=8
  Demux : Demux  Outputs=2
  Demux8 : Demux  Outputs=[2 1]
  Demux9 : Demux  Outputs=2
  EGM-96 Geoid Model : Subsystem  mask(EGM-96 geoid undulation model){}
      mask help: Computes the MSL (mean sea level) altitude as a function of position.
      mask init:
      | load('egm96');
      mask Help:
      | The block computes the mean-sea-level altitude relative to the WGS-84 geoid.
      | <P><B>Inputs:</B>
      | <LI>Position = the 3x1 vector of aircraft location [Latitude Longitude Altitude], in [rad rad m]</LI>
      | </P>
      | <P><B>Output:</B>
      | <LI>MSLAlt = the mean-sea-level altitude, in m</LI>
      | </P>
  Flat Earth to LLA : aerolibtransform2/Flat Earth to LLA  units=Metric (MKS)  ptype=Earth (WGS84)  F=1/298.257223563  R=6378137  LL0=FWFleet.IC.geodetic(1:2)  psi=0
  Gain : Gain  Gain=-1
  Ground Detection : Subsystem  mask(Ground detection){}
      mask help: Computes altitude above ground and sets a flag if AGL is negative.
      mask Help:
      | The block computes the altitude above ground (AGL) and sets a flag if the AGL is negative (used for ground contact detection).
      | <P><B>Inputs:</B>
      | <LI>MSLAlt = the altitude measured from mean-sea-level, in meters</LI>
      | <LI>GndAlt = the altitude of the terrain (above MSL) at current location, in meters</LI>
      | </P>
      | <P><B>Output:</B>
      | <LI>AConGnd = the aircraft-on-ground flag (0 if aircraft above ground, 1 if aircraft on the ground)</LI>
      | <LI>AGLAlt = the altitude of the aircraft above ground</LI>
      | </P>
  Ground Height : Constant  Value=Env.GroundAlt
  Ground Height1 : Constant  Value=Env.GroundAlt
  Latitude Bound [-180,180] : Subsystem
  Longitude Bound 0-360 : Subsystem  mask(Longitude bound){}
      mask help: Bounds the longitude to [0, 2pi]. When 0 bound is exceeded the longitude wraps back to 2pi; when the 2pi bound is exceeded the longitude wraps back to 0.
  Mux : Mux  Inputs=3
  README : simulink/Model-Wide Utilities/DocBlock  DocumentType=Text
      content=|
      | Navigation
      |
      | This block is library link that contains the navigational model and
      | equations. Included are equations relating the flat Earth position to
      | latitude/longitude, a simplified 2D table lookup version of the EGM-96
      | Geoid model for computation of MSL/AGL altitudes, and computation of
      | flight path and ground track angles.
  Saturation : Saturate  UpperLimit=Inf  LowerLimit=0
  Stop Simulation when A/C on the ground : Stop
  Trigonometric Function : Trigonometry  Operator=atan2
  Trigonometric Function1 : Trigonometry  Operator=atan2
  VecNorm : Subsystem
  Nav : Outport
  wires:
  Gain/1 -> Trigonometric Function/1
  Demux9/1 -> Trigonometric Function1/1
  Demux8/1 -> Demux9/1, VecNorm/1(I)
  Trigonometric Function1/1 -> Bus Creator1/7  "gndtrack [rad]"
  Demux9/2 -> Trigonometric Function1/2
  Trigonometric Function/1 -> Bus Creator1/8  "gamma [rad]"
  VecNorm/1(O) -> Trigonometric Function/2
  Demux8/2 -> Gain/1
  V_e [m/s]/1 -> Demux8/1
  Ground Detection/2(AGLAlt) -> Bus Creator1/6  "Alt (Above Ground Level) [m]"
  Saturation/1 -> Mux/3, Bus Creator1/3  "Altitude [m]"
  Ground Detection/1(AConGnd) -> Stop Simulation when A/C on the ground/1, Bus Creator1/5  "AC on Ground"
  Ground Height1/1 -> Ground Detection/2(GndAlt)
  EGM-96 Geoid Model/1(MSLAlt) -> Bus Creator1/4, Ground Detection/1(MSLAlt)  "Alt (Above Mean Sea Level) [m]"
  Bus Creator1/1 -> Nav/1
  Ground Height/1 -> Flat Earth to LLA/2
  X_e [m]/1 -> Flat Earth to LLA/1
  Demux/2 -> Longitude Bound 0-360/1(In), Bus Creator1/2  "Geodetic Longitude [deg]"
  Demux/1 -> Bus Creator1/1, Latitude Bound [-180,180]/1(In)  "Geodetic Latitude [deg]"
  Flat Earth to LLA/2 -> Saturation/1  "Altitude [m]"
  Flat Earth to LLA/1 -> Demux/1
  Mux/1 -> EGM-96 Geoid Model/1(Position)
  Longitude Bound 0-360/1(Out) -> Mux/2
  Latitude Bound [-180,180]/1(Out) -> Mux/1

== system MultiVehicleModel/Reconnaissance Fleet/UMN - Uninhabited Aerial Vehicle Fleet/Nonlinear UAV Model/Environment/Magnetic Model ==
  Altitude : Inport
  Latitude : Inport  Port=2
  Longitude : Inport  Port=3
  Decimal Year : Inport  Port=4
  WMM 2005 : aerolibobsolete/World Magnetic Model 2005  units=Metric (MKS)  time_in=off  month=August  day=1  year=2009  action=None  h_out=off  dec_out=off  inc_out=off  ti_out=off
  term4 : Terminator
  Magnetic Field : Outport
  wires:
  Altitude/1 -> WMM 2005/1
  Latitude/1 -> WMM 2005/2
  Longitude/1 -> WMM 2005/3
  WMM 2005/1 -> Magnetic Field/1
  Decimal Year/1 -> term4/1

== system MultiVehicleModel/Reconnaissance Fleet/UMN - Uninhabited Aerial Vehicle Fleet/Nonlinear UAV Model/Environment/Winds ==
  V_s [m/s] : Inport
  R_be [3x3] : Inport  Port=2
  h (m) : Inport  Port=3
  Wind & Turbulence : Environment_Lib/Wind & Turbulence
  SteadyWind [m/s] : Outport
  WindGust [m/s] : Outport  Port=2
  WindAngVel [rad/s] : Outport  Port=3
  wires:
  V_s [m/s]/1 -> Wind & Turbulence/1
  R_be [3x3]/1 -> Wind & Turbulence/2
  h (m)/1 -> Wind & Turbulence/3
  Wind & Turbulence/1 -> SteadyWind [m/s]/1
  Wind & Turbulence/2 -> WindGust [m/s]/1
  Wind & Turbulence/3 -> WindAngVel [rad/s]/1

== system MultiVehicleModel/Reconnaissance Fleet/UMN - Uninhabited Aerial Vehicle Fleet/Nonlinear UAV Model/Forces and Moments/Aerodynamic Forces and Moments ==
  Control Surfaces : Inport
  States : Inport  Port=2
  EnvData : Inport  Port=3
  Bus Selector : BusSelector  OutputSignals=Density [kg/m^3]
  Bus Selector1 : BusSelector  OutputSignals=V_b [m/s]
  CG Position : Constant  Value=AC.Geometry.rCG
  CP Position : Constant  Value=AC.Geometry.AeroCenter
  Dynamic Pressure : aerolibasang/Dynamic Pressure
  "Forces and Moments Calculation " : aerolibadyn/Aerodynamic Forces and Moments   inputAxes=Wind  outputForceAxes=Body  outputMomentAxes=Wind  S=AC.Geometry.S  b=AC.Geometry.b  cbar=AC.Geometry.c
  Ultrastick : Ultrastick_Aero_Lib/Ultrastick
  M_aero_body : Outport
  F_aero_body : Outport  Port=2
  wires:
  Control Surfaces/1 -> Ultrastick/1
  Dynamic Pressure/1 -> "Forces and Moments Calculation "/2
  "Forces and Moments Calculation "/2 -> M_aero_body/1
  "Forces and Moments Calculation "/1 -> F_aero_body/1
  Bus Selector/1 -> Dynamic Pressure/2  "<Density [kg/m^3]>"
  States/1 -> Ultrastick/2, Bus Selector1/1
  EnvData/1 -> Bus Selector/1
  CP Position/1 -> "Forces and Moments Calculation "/4
  CG Position/1 -> "Forces and Moments Calculation "/3
  Ultrastick/1 -> "Forces and Moments Calculation "/1
  Bus Selector1/1 -> Dynamic Pressure/1, "Forces and Moments Calculation "/5  "<V_b [m/s]>"

== system MultiVehicleModel/Reconnaissance Fleet/UMN - Uninhabited Aerial Vehicle Fleet/Control System/Control_Algorithm /Altitude Tracker/Altitude Tracker ==
  " h_out" : Inport
  error : Inport  Port=2
  Anti Windup : Actuator_Lib/Anti Windup  MAX_DEF=AC.Actuator.elevator.PosLim-TrimCondition.Inputs.elevator  MIN_DEF=AC.Actuator.elevator.NegLim-TrimCondition.Inputs.elevator  gain_sign=on
  Discrete-Time Integrator : DiscreteIntegrator  SampleTime=.02  ICPrevOutput=DiscIntNeverNeededParam  ICPrevScaledInput=DiscIntNeverNeededParam
  Gain : Gain  Gain=control.kp_AT
  Gain1 : Gain  Gain=control.ki_AT
  Sum : Sum  Inputs=|++
  h_out : Outport
  wires:
  Discrete-Time Integrator/1 -> Gain1/1
  Gain1/1 -> Sum/1
  Sum/1 -> h_out/1
  Gain/1 -> Sum/2
  " h_out"/1 -> Anti Windup/1
  error/1 -> Anti Windup/2, Gain/1
  Anti Windup/1 -> Discrete-Time Integrator/1

== system MultiVehicleModel/Reconnaissance Fleet/UMN - Uninhabited Aerial Vehicle Fleet/Control System/Control_Algorithm /baseline control/Phi Tracker ==
  phi_cmd [rad] : Inport
  phi [rad] : Inport  Port=2
  p [rad] : Inport  Port=3
  Gain1 : Gain  Gain=roll_gains(3)
  Phi Trim : Constant  Value=TrimCondition.AttitudeIni(1)
  Roll Tracker : Subsystem
  Saturation1 : Saturate  UpperLimit=AC.Actuator.r_aileron.PosLim-TrimCondition.Inputs.r_aileron  LowerLimit=AC.Actuator.r_aileron.NegLim-TrimCondition.Inputs.r_aileron  SampleTime=SampleTime
  Sum2 : Sum  Inputs=|+-  SampleTime=SampleTime
  Sum3 : Sum  Inputs=|+-  SampleTime=SampleTime
  Sum5 : Sum  Inputs=|+-  SampleTime=SampleTime
  aileron [rad] : Outport
  wires:
  Roll Tracker/1(aileron) -> Sum3/1
  Saturation1/1 -> aileron [rad]/1
  phi [rad]/1 -> Sum5/1
  Sum5/1 -> Sum2/2
  Phi Trim/1 -> Sum5/2
  Sum2/1 -> Roll Tracker/2(error)
  Sum3/1 -> Roll Tracker/1(aileron cmd), Saturation1/1
  p [rad]/1 -> Gain1/1
  Gain1/1 -> Sum3/2
  phi_cmd [rad]/1 -> Sum2/1

== system MultiVehicleModel/Reconnaissance Fleet/UMN - Uninhabited Aerial Vehicle Fleet/Control System/Control_Algorithm /baseline control/Theta Tracker ==
  theta_cmd [rad/s] : Inport
  theta [rad] : Inport  Port=2
  q [rad/sec] : Inport  Port=3
  " Theta Trim" : Constant  Value=TrimCondition.AttitudeIni(2)
  Gain1 : Gain  Gain=pitch_gains(3)
  Pitch Tracker : Subsystem
  Saturation1 : Saturate  UpperLimit=AC.Actuator.elevator.PosLim-TrimCondition.Inputs.elevator  LowerLimit=AC.Actuator.elevator.NegLim-TrimCondition.Inputs.elevator  SampleTime=SampleTime
  Sum : Sum  Inputs=|+-  SampleTime=SampleTime
  Sum1 : Sum  Inputs=|+-  SampleTime=SampleTime
  Sum2 : Sum  Inputs=|+-  SampleTime=SampleTime
  elevator [rad] : Outport
  wires:
  Sum2/1 -> Pitch Tracker/2(error)
  Saturation1/1 -> elevator [rad]/1
  Sum1/1 -> Sum2/2
  " Theta Trim"/1 -> Sum1/2
  theta [rad]/1 -> Sum1/1
  theta_cmd [rad/s]/1 -> Sum2/1
  Pitch Tracker/1(pitch_out) -> Sum/1
  Sum/1 -> Pitch Tracker/1(eleveator cmd), Saturation1/1
  q [rad/sec]/1 -> Gain1/1
  Gain1/1 -> Sum/2

== system MultiVehicleModel/Reconnaissance Fleet/UMN - Uninhabited Aerial Vehicle Fleet/Control System/Control_Algorithm /baseline control/Yaw Damper ==
  r [rad/sec] : Inport
  Discrete Transfer Fcn : DiscreteTransferFcn  Numerator=yaw_damper_num  Denominator=yaw_damper_den  SampleTime=SampleTime
  rudder [rad] : Outport
  wires:
  Discrete Transfer Fcn/1 -> rudder [rad]/1
  r [rad/sec]/1 -> Discrete Transfer Fcn/1

== system MultiVehicleModel/Reconnaissance Fleet/UMN - Uninhabited Aerial Vehicle Fleet/Nonlinear UAV Model/Auxiliary Equations/Euler Angle Bounds/2pi Bound ==
  In : Inport
  2pi : Constant  Value=2*pi
  Math Function : Math  Operator=mod  SaturateOnIntegerOverflow=on
  Out : Outport
  wires:
  In/1 -> Math Function/1
  2pi/1 -> Math Function/2
  Math Function/1 -> Out/1

== system MultiVehicleModel/Reconnaissance Fleet/UMN - Uninhabited Aerial Vehicle Fleet/Nonlinear UAV Model/Auxiliary Equations/Euler Angle Bounds/pi Bound ==
  In : Inport
  Math Function : Math  Operator=mod  SaturateOnIntegerOverflow=on
  Sum1 : Sum  Inputs=|+-  SaturateOnIntegerOverflow=on  InputSameDT=on  OutDataTypeStr=Inherit: Same as first input
  Sum2 : Sum  Inputs=|++  SaturateOnIntegerOverflow=on  InputSameDT=on  OutDataTypeStr=Inherit: Same as first input
  pi : Constant  Value=pi
  pi1 : Constant  Value=2*pi
  Out : Outport
  wires:
  Sum1/1 -> Out/1
  pi/1 -> Sum1/2, Sum2/2
  Sum2/1 -> Math Function/1
  In/1 -> Sum2/1
  pi1/1 -> Math Function/2
  Math Function/1 -> Sum1/1

== system MultiVehicleModel/Reconnaissance Fleet/UMN - Uninhabited Aerial Vehicle Fleet/Nonlinear UAV Model/Auxiliary Equations/Euler Angle Bounds/pi//2 Bound ==
  In : Inport
  Math Function : Math  Operator=mod  SaturateOnIntegerOverflow=on
  Sum1 : Sum  Inputs=|+-  SaturateOnIntegerOverflow=on  InputSameDT=on  OutDataTypeStr=Inherit: Same as first input
  Sum2 : Sum  Inputs=|++  SaturateOnIntegerOverflow=on  InputSameDT=on  OutDataTypeStr=Inherit: Same as first input
  pi : Constant  Value=pi/2
  pi1 : Constant  Value=pi
  Out : Outport
  wires:
  Math Function/1 -> Sum1/1
  pi1/1 -> Math Function/2
  In/1 -> Sum2/1
  Sum2/1 -> Math Function/1
  pi/1 -> Sum2/2, Sum1/2
  Sum1/1 -> Out/1

== system MultiVehicleModel/Reconnaissance Fleet/UMN - Uninhabited Aerial Vehicle Fleet/Nonlinear UAV Model/Auxiliary Equations/Navigation/EGM-96 Geoid Model ==
  Position : Inport
  Demux2 : Demux  Outputs=3
  Look-Up Table (2-D) : Lookup2D  RowIndex=Lat  ColumnIndex=Lon  Table=Alterr'  SaturateOnIntegerOverflow=on  InputSameDT=on
  Sum : Sum  Inputs=|+++
  WGS-84 correction : Constant  Value=-0.53
  MSLAlt : Outport
  wires:
  Demux2/2 -> Look-Up Table (2-D)/2
  Demux2/1 -> Look-Up Table (2-D)/1
  Position/1 -> Demux2/1
  Demux2/3 -> Sum/2
  Sum/1 -> MSLAlt/1
  Look-Up Table (2-D)/1 -> Sum/1
  WGS-84 correction/1 -> Sum/3

== system MultiVehicleModel/Reconnaissance Fleet/UMN - Uninhabited Aerial Vehicle Fleet/Nonlinear UAV Model/Auxiliary Equations/Navigation/Ground Detection ==
  MSLAlt : Inport
  GndAlt : Inport  Port=2
  False : Constant  Value=0
  Sum : Sum  Inputs=|+-  SaturateOnIntegerOverflow=on  InputSameDT=on  OutDataTypeStr=Inherit: Same as first input
  Switch : Switch  SaturateOnIntegerOverflow=on  InputSameDT=on
  True : Constant
  AConGnd : Outport
  AGLAlt : Outport  Port=2
  wires:
  MSLAlt/1 -> Sum/1
  GndAlt/1 -> Sum/2
  Sum/1 -> Switch/2, AGLAlt/1
  False/1 -> Switch/1
  True/1 -> Switch/3
  Switch/1 -> AConGnd/1

== system MultiVehicleModel/Reconnaissance Fleet/UMN - Uninhabited Aerial Vehicle Fleet/Nonlinear UAV Model/Auxiliary Equations/Navigation/Latitude Bound [-180,180] ==
  In : Inport
  2pi : Constant  Value=360
  Math Function : Math  Operator=mod  SaturateOnIntegerOverflow=on
  Sum1 : Sum  Inputs=|+-  SaturateOnIntegerOverflow=on  InputSameDT=on  OutDataTypeStr=Inherit: Same as first input
  Sum2 : Sum  Inputs=|++  SaturateOnIntegerOverflow=on  InputSameDT=on  OutDataTypeStr=Inherit: Same as first input
  pi : Constant  Value=180
  Out : Outport
  wires:
  Math Function/1 -> Sum1/1
  2pi/1 -> Math Function/2
  In/1 -> Sum2/1
  Sum2/1 -> Math Function/1
  pi/1 -> Sum2/2, Sum1/2
  Sum1/1 -> Out/1

== system MultiVehicleModel/Reconnaissance Fleet/UMN - Uninhabited Aerial Vehicle Fleet/Nonlinear UAV Model/Auxiliary Equations/Navigation/Longitude Bound 0-360 ==
  In : Inport
  2pi : Constant  Value=360
  Math Function : Math  Operator=mod  SaturateOnIntegerOverflow=on
  Out : Outport
  wires:
  Math Function/1 -> Out/1
  2pi/1 -> Math Function/2
  In/1 -> Math Function/1

== system MultiVehicleModel/Reconnaissance Fleet/UMN - Uninhabited Aerial Vehicle Fleet/Nonlinear UAV Model/Auxiliary Equations/Navigation/VecNorm ==
  I : Inport
  Math Function2 : Math  Operator=sqrt  SaturateOnIntegerOverflow=on
  Product : Product  RndMeth=Zero
  Sum of Elements : Sum  Inputs=+
  O : Outport
  wires:
  Sum of Elements/1 -> Math Function2/1
  Product/1 -> Sum of Elements/1
  I/1 -> Product/2, Product/1
  Math Function2/1 -> O/1

== system MultiVehicleModel/Reconnaissance Fleet/UMN - Uninhabited Aerial Vehicle Fleet/Control System/Control_Algorithm /baseline control/Phi Tracker/Roll Tracker ==
  aileron cmd : Inport
  error : Inport  Port=2
  Anti Windup : Actuator_Lib/Anti Windup  MAX_DEF=AC.Actuator.r_aileron.PosLim-TrimCondition.Inputs.r_aileron  MIN_DEF=AC.Actuator.r_aileron.NegLim-TrimCondition.Inputs.r_aileron  gain_sign=off
  Discrete-Time Integrator : DiscreteIntegrator  SampleTime=.02  ICPrevOutput=DiscIntNeverNeededParam  ICPrevScaledInput=DiscIntNeverNeededParam
  Gain : Gain  Gain=roll_gains(1)  SampleTime=SampleTime
  Gain1 : Gain  Gain=roll_gains(2)  SampleTime=SampleTime
  Sum : Sum  Inputs=|++  SampleTime=.02
  aileron : Outport
  wires:
  Anti Windup/1 -> Discrete-Time Integrator/1
  aileron cmd/1 -> Anti Windup/1
  error/1 -> Anti Windup/2, Gain/1
  Gain/1 -> Sum/2
  Sum/1 -> aileron/1
  Gain1/1 -> Sum/1
  Discrete-Time Integrator/1 -> Gain1/1

== system MultiVehicleModel/Reconnaissance Fleet/UMN - Uninhabited Aerial Vehicle Fleet/Control System/Control_Algorithm /baseline control/Theta Tracker/Pitch Tracker ==
  eleveator cmd : Inport
  error : Inport  Port=2
  Anti Windup : Actuator_Lib/Anti Windup  MAX_DEF=AC.Actuator.elevator.PosLim-TrimCondition.Inputs.elevator-15*pi/180  MIN_DEF=AC.Actuator.elevator.NegLim-TrimCondition.Inputs.elevator+15*pi/180  gain_sign=off
  Discrete-Time Integrator : DiscreteIntegrator  SampleTime=.02  ICPrevOutput=DiscIntNeverNeededParam  ICPrevScaledInput=DiscIntNeverNeededParam
  Gain : Gain  Gain=pitch_gains(1)
  Gain1 : Gain  Gain=pitch_gains(2)
  Sum : Sum  Inputs=|++
  pitch_out : Outport
  wires:
  eleveator cmd/1 -> Anti Windup/1
  Anti Windup/1 -> Discrete-Time Integrator/1
  error/1 -> Anti Windup/2, Gain/1
  Gain/1 -> Sum/2
  Sum/1 -> pitch_out/1
  Gain1/1 -> Sum/1
  Discrete-Time Integrator/1 -> Gain1/1

== matlab function MultiVehicleModel/Reconnaissance Fleet/UMN - Uninhabited Aerial Vehicle Fleet/Guidance algorithm/Ground track angle computation based on waypoints ==
  data: hCmd output; waypoint input; psi input; Pned input; psiTarget output; fcn input
function [hCmd ,psiTarget]     = fcn(waypoint, psi, Pned, fcn )
%#codegen
psiErrorMax = 90*pi/180; 
RTurnMin = 150; 

nPoints = size(waypoint, 2) ;

%size(waypoint)
% persitent variable used to keep trak of next waypoint
persistent wpointer; 

% persitent variable used to keep track of operation mode. 
% mode = 1: tracking next waypoint
% mode = 2: tracking an intermediate waypoint to guarantee 
persistent mode; 

% auxilary waypoint coordinates for operation in mode 2
persistent wpointAux; 

if isempty(wpointer) 
wpointer = 1; 
end

if isempty(mode) 
mode = 1; 
end

if isempty(wpointAux) 
wpointAux = zeros(2, 2);  
end

psiTarget =0;


switch  fcn
    case 1
        wpointer  = 1;
        disp('resetting mission ... ')
    otherwise
end

%waypoint(:, wpointer)

% a waypoint is reached if the distance to the aircraft is less than 20 m
if (mode ==1 && norm(Pned(1:2) - waypoint(1:2, wpointer) )< 10 ) 
    if(wpointer ~= nPoints)        
      
        psiTarget = atan2( waypoint(2,wpointer+1) - Pned(2) , waypoint(1,wpointer+1) - Pned(1)) ;
        % psiTarget from 0 to 360 deg only
        if (psiTarget <0)
            psiTarget = 2*pi+psiTarget ; 
        end
        
        psiError = psiTarget - psi; 

        if (psiError < -pi)
           psiError = 2*pi+psiError ; 
        end

        if (psiError > pi)
            psiError = -2*pi+psiError ; 
        end
        
        
        if ( abs(psiError) > psiErrorMax)
            mode = 2;
            % after intermediate waypoint we will pass through the last
            % waypoint

            psiAux = psiTarget - pi; 
            wpointAux(1,1) = Pned(1)+  RTurnMin*cos(psiAux) ; 
            wpointAux(2,1) = Pned(2)+  RTurnMin*sin(psiAux) ; 
            
            wpointAux(1,2) = Pned(1)+  RTurnMin*cos(psiAux)/2 ; 
            wpointAux(2,2) = Pned(2)+  RTurnMin*sin(psiAux)/2 ; 
            
            %disp('aux wpoint')
            %wpointAux
            %disp('my pos')
            %Pned(1:2);
            
            %disp('psi')
            %psi
            
            %disp('psi trget')
            %psiTarget
            
            
            
        else
            wpointer = wpointer + 1 ;
        end

        %{
        if (psiError < -pi)
            psiError = 2*pi+psiError ; 
        end

        if (psiError > pi)
            psiError = -2*pi+psiError ; 
        end
        %}
        
    end
    
    
end

if (mode ==2 && norm(Pned(1:2) - wpointAux (:,1) )< 10)

    mode =3 ; 
    
    %disp('aux mode 2 completed')
end

if (mode ==3 && norm(Pned(1:2) - wpointAux (:,2) )< 10)

    mode =1 ; 
    
    %disp('aux mode 3 completed')
end


if mode ==1 
% computing the angle between the vehicle ground velocity vector and vector
% connecting thevehicle body frame and waypoint
psiTarget = atan2( waypoint(2,wpointer) - Pned(2) , waypoint(1,wpointer) - Pned(1)) ;
end

if mode ==2
  psiTarget = atan2( wpointAux(2,1) - Pned(2) , wpointAux(1,1) - Pned(1)) ;
end

if mode ==3
  psiTarget = atan2( wpointAux(2,2) - Pned(2) , wpointAux(1,2) - Pned(1)) ;
end


% psiTarget from 0 to 360 deg only
if (psiTarget <0)
    psiTarget = 2*pi+psiTarget ; 
end

hCmd  =  waypoint(3,wpointer) ;

 %waypoint(:,wpointer) 

%[xNorth, yEast, zDown] = geodetic2ned(waypoint(1,wpointer), waypoint(2,wpointer) , waypoint(2,wpointer) , 0, 0, 0) ;

== matlab function MultiVehicleModel/Mission planning and monitoring - Network/Mission Plan Generation for fixed wing UAV fleet Runs on the server // cloud /Fleet Waypoint Reading from UDP/DataBase  ==
  data: uavID input; functionID input; dataUAV input; dataFleet output; fcnFleet output; status input; nAC parameter double size=[1,1]; LLA0 input
function [dataFleet,fcnFleet] = fcn(uavID, functionID , dataUAV, status, nAC, LLA0)
%#codegen

nWPs = 100; % maximum number of waypoints
fcnFleet = zeros(nAC,1) ;

persistent waypointsFleet; 

if isempty(waypointsFleet)
    waypointsFleet = zeros(3,nWPs, nAC);  
    waypointsFleet(1,:,:) = ones(1,nWPs, nAC)*LLA0(1) ; 
    waypointsFleet(2,:,:) = ones(1,nWPs, nAC)*LLA0(2) ; 
    waypointsFleet(3,:,:) = ones(1,nWPs, nAC)*LLA0(3) ; 
end

switch functionID
    case 1 % setting waypoint list of a UAV into database
        if (uavID <= nAC )
            waypointsFleet(:,1:nWPs,uavID) = reshape(dataUAV, 3 ,nWPs  ); 
            if status ==1
                fcnFleet(uavID) =functionID ; % reset
                disp('status = 1') ;
            end
        end
        
        
    otherwise
        
        
    
end


dataFleet = waypointsFleet(1:3,:,:);

== matlab function MultiVehicleModel/Reconnaissance Fleet/UMN - Uninhabited Aerial Vehicle Fleet/Control System/Control_Algorithm /ground trak angle control law/normalize angle between pi and -pi (rad) ==
  data: angleOut output; angleIn input
function angleOut    = fcn(angleIn)
%#codegen
angleOut = angleIn;
if (angleOut < -pi)
   angleOut = 2*pi+angleOut ; 
end

if (angleOut > pi)
    angleOut = -2*pi+angleOut ; 
end

== matlab function MultiVehicleModel/Mission planning and monitoring - Network/Mission Plan Generation for rotorcraft fleet Runs on the server // cloud/Fleet Waypoint Reading from UDP/DataBase  ==
  data: uavID input; functionID input; dataUAV input; dataWP output; dataHT output; fcnFleet output; status input; nAC parameter double size=[1,1]; LLA0 input
function [dataWP, dataHT,fcnFleet] = fcn(uavID, functionID , dataUAV, status, nAC, LLA0 )
%#codegen

nWPs = 100; % maximum number of waypoints
fcnFleet = zeros(nAC,1) ;
dimWP =5; 
persistent waypointsFleet; 

if isempty(waypointsFleet)
    waypointsFleet = zeros(dimWP,nWPs, nAC);  
    waypointsFleet(1,:,:) = ones(1,nWPs, nAC)*LLA0(1); 
    waypointsFleet(2,:,:) = ones(1,nWPs, nAC)*LLA0(2); 
    waypointsFleet(3,:,:) = ones(1,nWPs, nAC)*LLA0(3); 
end

switch functionID
    case 1 % setting waypoint list of a UAV into database
        if (uavID <= nAC )
            waypointsFleet(:,1:nWPs,uavID) = reshape(dataUAV, dimWP ,nWPs  ) ; 
            if status ==1
                fcnFleet(uavID) =functionID ; % reset
                disp('status = 1') ;
                %waypointsFleet 
            end
        end
        
        
    otherwise
        
        
    
end


%dataFleet = waypointsFleet(1:dimWP,:,:);
dataWP = waypointsFleet(1:3,:,:);
dataHT = waypointsFleet(4:5,:,:);

== matlab function MultiVehicleModel/Rotorcraft fleet/Multiple Rotorcraft/vehicle controller1/MATLAB Function ==
  data: Vec_b input; UnitVec_xy output; psi input
function UnitVec_xy = fcn(Vec_b , psi)
%#codegen
T = [cos(psi) sin(psi) ; -sin(psi) cos(psi)] ; 
UnitVec_xy = T*Vec_b; 

%{
if norm(UnitVec_xy) > 0.2
    UnitVec_xy = UnitVec_xy/norm(UnitVec_xy) ;
else
    UnitVec_xy = [0; 0] ;
end
%}
